simulink model "SchemeWith2DCMachine"  (R2021b)
settings: Solver=VariableStepAuto  StartTime=0.0  StopTime=10  RelTol=1e-3
libraries: spsDiodeLib x7, spsVoltageMeasurementLib x3, spsDCMachineLib x2, spsMeanLib x2, spsSeriesRLCBranchLib x2, spsDCVoltageSourceLib x1, spsGroundLib x1, spsMosfetLib x1, spsThreePhaseSourceLib x1, spspowerguiLib x1
settings Model: Creator=kkaya674  LastModifiedBy=kkaya674

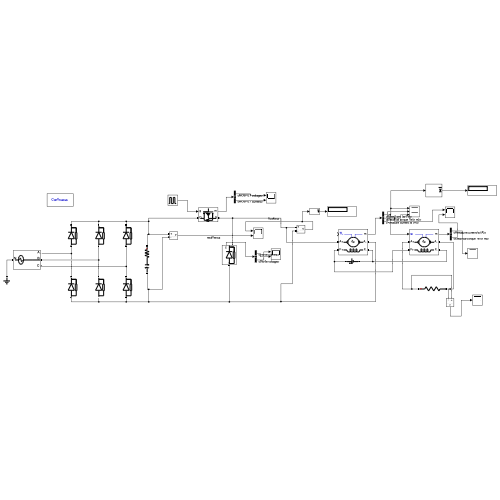
[thumbnail: Simulink's stored preview of the top-level diagram]
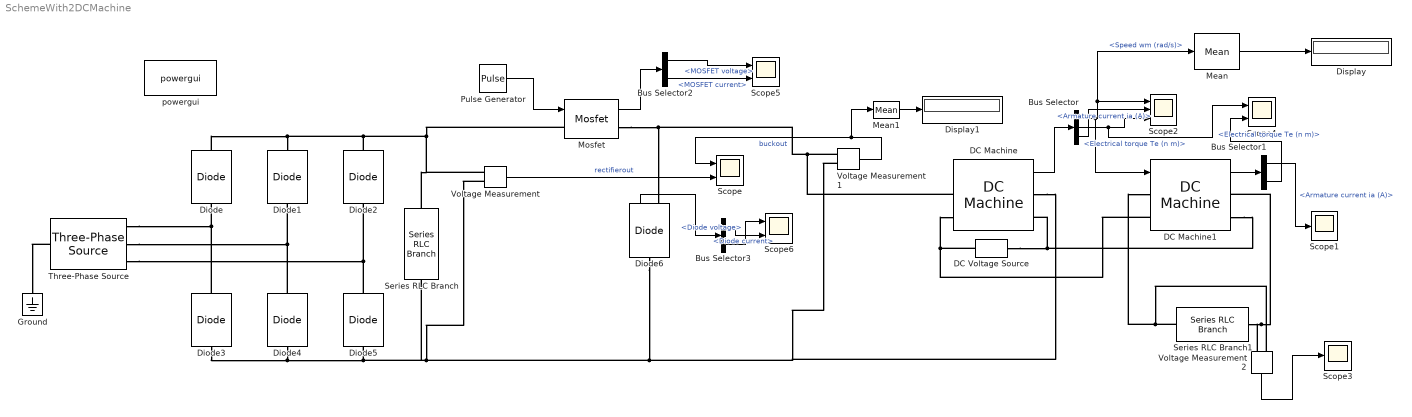
== system SchemeWith2DCMachine ==
  Bus Selector : BusSelector  OutputSignals=Speed wm (rad/s),Electrical torque Te (n m),Armature current ia (A)
  Bus Selector1 : BusSelector  OutputSignals=Armature current ia (A),Electrical torque Te (n m)
  Bus Selector2 : BusSelector  OutputSignals=MOSFET voltage,MOSFET current
  Bus Selector3 : BusSelector  OutputSignals=Diode current,Diode voltage
  DC Machine : spsDCMachineLib/DC Machine  PresetModel=03: 5HP 500V 1750RPM Field:300V  MechanicalLoad=Torque TL  FieldType=Wound  ShowDetailedParameters=on  MeasurementBus=off  RLa=[11.2 0.1215]  RLf=[281.2 156]  Laf=1.976  MachineConstant=Torque constant (N.m/A)  Ke=1.8  Kt=1.8  J=0.02215  Bm=0.002953  Tf=0.5161  w0=120  Ifinit=1.06685632871799  TsPowergui=0  TsBlock=-1
  DC Machine1 : spsDCMachineLib/DC Machine  PresetModel=03: 5HP 500V 1750RPM Field:300V  MechanicalLoad=Speed w  FieldType=Wound  ShowDetailedParameters=on  MeasurementBus=off  RLa=[11.2 0.1215]  RLf=[281.2 156]  Laf=1.976  MachineConstant=Torque constant (N.m/A)  Ke=1.8  Kt=1.8  J=0.02215  Bm=0.002953  Tf=0.5161  w0=1  Ifinit=1.06685632871799  TsPowergui=0  TsBlock=-1
  DC Voltage Source : spsDCVoltageSourceLib/DC Voltage Source  Amplitude=300  Measurements=None
  Diode{,1..5} (6 alike) : spsDiodeLib/Diode  Ron=0.001  Lon=0  Vf=0.8  IC=0  UseSnubber=0  Rs=500  Cs=250e-9  Measurements=off
  Diode6 : spsDiodeLib/Diode  Ron=0.001  Lon=0  Vf=0.8  IC=0  UseSnubber=0  Rs=500  Cs=250e-9  Measurements=on
  Display : Display
  Display1 : Display
  Ground : spsGroundLib/Ground  LConnTagsString=a
  Mean : spsMeanLib/Mean  Freq=60  Vinit=0  Ts=0
  Mean1 : spsMeanLib/Mean  Freq=60  Vinit=0  Ts=0
  Mosfet : spsMosfetLib/Mosfet  Ron=0.1  Lon=0  Rd=0.01  Vfd=0  IC=0  Rs=1e5  Cs=inf  Measurements=on
  Pulse Generator : DiscretePulseGenerator  PulseType=Time based  Period=0.02  PulseWidth=0.5  VectorParams1D=off
  Scope{,4..6} (4 alike) : Scope  NumInputPorts=2
  Scope1 : Scope
  Scope2 : Scope  NumInputPorts=3
  Scope3 : Scope
  Series RLC Branch : spsSeriesRLCBranchLib/Series RLC Branch  LConnTagsString=__new0  RConnTagsString=__new0  BranchType=RC  Resistance=100  Inductance=1e-3  SetiL0=off  InitialCurrent=0  Capacitance=1e-6  Setx0=off  InitialVoltage=0  Measurements=None
  Series RLC Branch1 : spsSeriesRLCBranchLib/Series RLC Branch  LConnTagsString=__new0  RConnTagsString=__new0  BranchType=R  Resistance=192  Inductance=1e-3  SetiL0=off  InitialCurrent=0  Capacitance=1e-6  Setx0=off  InitialVoltage=0  Measurements=None
  Three-Phase Source : spsThreePhaseSourceLib/Three-Phase Source  InternalConnection=Yn  VoltagePhases=off  Voltage=400  PhaseAngle=0  Voltage_phases=[25e3 25e3 25e3]/sqrt(3)  PhaseAngles_phases=[0 -120 +120]  Frequency=50  NonIdealSource=off  SpecifyImpedance=off  Resistance=0.8929  Inductance=16.58e-3  ShortCircuitLevel=100e6  BaseVoltage=25e3  XRratio=7  BusType=swing  Pref=10e3  Qref=0  Prefabc=[10e3, 10e3, 10e3]  Qrefabc=[0, 0, 0]  Qmin=-inf  Qmax=inf
  Voltage Measurement : spsVoltageMeasurementLib/Voltage Measurement  PhasorSimulation=off  OutputType=Complex  PSBequivalent=0
  Voltage Measurement1 : spsVoltageMeasurementLib/Voltage Measurement  PhasorSimulation=off  OutputType=Complex  PSBequivalent=0
  Voltage Measurement2 : spsVoltageMeasurementLib/Voltage Measurement  PhasorSimulation=off  OutputType=Complex  PSBequivalent=0
  powergui : spspowerguiLib/powergui  Priority=1  SimulationMode=Continuous  SampleTime=50e-6  frequency=60  Iterations=50  frequencyindice=0  Pbase=100e6  ErrMax=1e-4  UnitsV=kV  UnitsW=MW  buscounter=0  FunctionMessages=off  echomessages=off  EnableUseOfTLC=off  CurrentSourceSwitches=off  DisableSnubberDevices=off  DisableRonSwitches=off  DisableVfSwitches=off  DisplayEquations=off  AutomaticDiscreteSolvers=off  SolverType=Tustin/Backward Euler (TBE)  Interpol=off  ExternalGateDelay=off  methode=off  Ts=100  x0status=blocks  SPID=on  SwTol=0  HookPort=off  NonlinearTolerance=1e-4  nMaxIteration=100  ContinueOnMaxIteration=off  RestoreLinks=warning  ResistiveCurrentMeasurement=off  Frange=[0:2:500]  Ylog=off  Xlog=on  ShowGrid=off  save=off  variable=ZData  structure=0  ZoomFFT=off  StartTime=0.0  cycles=1  DisplayStyle=1  fundamental=60  FreqAxis=off  MaxFrequency=1000  frequencyindicesteady=1  RmsSteady=1  display=off
  wires:
  Voltage Measurement/1 -> Scope/2  "rectifierout"
  Pulse Generator/1 -> Mosfet/1
  Voltage Measurement1/1 -> Mean1/1, Scope/1  "buckout"
  DC Machine/1 -> Bus Selector/1
  Bus Selector/1 -> DC Machine1/1, Scope2/1, Mean/1  "<Speed wm (rad/s)>"
  DC Machine1/1 -> Bus Selector1/1
  Bus Selector1/1 -> Scope1/1  "<Armature current ia (A)>"
  Mean/1 -> Display/1
  Voltage Measurement2/1 -> Scope3/1
  Mean1/1 -> Display1/1
  Bus Selector/2 -> Scope4/1, Scope2/3  "<Electrical torque Te (n m)>"
  Bus Selector/3 -> Scope2/2  "<Armature current ia (A)>"
  Bus Selector1/2 -> Scope4/2  "<Electrical torque Te (n m)>"
  Mosfet/1 -> Bus Selector2/1
  Bus Selector2/1 -> Scope5/1  "<MOSFET voltage>"
  Bus Selector2/2 -> Scope5/2  "<MOSFET current>"
  Diode6/1 -> Bus Selector3/1
  Bus Selector3/1 -> Scope6/2  "<Diode current>"
  Bus Selector3/2 -> Scope6/1  "<Diode voltage>"
  connections:
  Three-Phase Source/RConn1 -- Diode/LConn1 -- Diode3/RConn1
  Three-Phase Source/RConn2 -- Diode1/LConn1 -- Diode4/RConn1
  Three-Phase Source/RConn3 -- Diode5/RConn1 -- Diode2/LConn1
  Diode4/LConn1 -- Diode3/LConn1 -- Series RLC Branch/RConn1 -- Voltage Measurement/LConn2 -- Voltage Measurement1/LConn2 -- DC Machine/RConn1 -- Diode6/LConn1 -- Diode5/LConn1
  Diode/RConn1 -- Mosfet/LConn1 -- Series RLC Branch/LConn1 -- Voltage Measurement/LConn1 -- Diode2/RConn1 -- Diode1/RConn1
  Three-Phase Source/LConn1 -- Ground/LConn1
  DC Voltage Source/RConn1 -- DC Machine1/LConn2 -- DC Machine/LConn2
  DC Voltage Source/LConn1 -- DC Machine1/RConn2 -- DC Machine/RConn2
  Series RLC Branch1/LConn1 -- DC Machine1/LConn1 -- Voltage Measurement2/LConn1
  Series RLC Branch1/RConn1 -- DC Machine1/RConn1 -- Voltage Measurement2/LConn2
  Voltage Measurement1/LConn1 -- DC Machine/LConn1 -- Mosfet/RConn1 -- Diode6/RConn1
